simulink model "BALL_BALACING"  (R2021a)
settings: Solver=FixedStepAuto  StartTime=0.0  StopTime=10.0  RelTol=1e-3  EnableMultiTasking=on
libraries: arduinosensorlib x1, arduinolib x1
settings Model: SILPILModeSetting=veronly  ExtModeTrigDuration=2  Creator=Waseem Sajjad  LastModifiedBy=Waseem Sajjad
settings OptimizationCC: EnhancedBackFolding=on  PassReuseOutputArgsAs=Individual arguments  ZeroExternalMemoryAtStartup=off  ZeroInternalMemoryAtStartup=off  MaxStackSize=64  OptimizeBlockOrder=speed  DifferentSizesBufferReuse=on  OptimizationCustomize=off  EfficientTunableParamExpr=on
settings DebuggingCC: ParameterTunabilityLossMsg=error
settings HardwareCC: ProdBitPerInt=16  ProdBitPerPointer=16  ProdBitPerSizeT=16  ProdBitPerPtrDiffT=16  ProdLargestAtomicFloat=None  ProdWordSize=8  ProdHWDeviceType=Atmel->AVR
settings SFSimCC: MATLABDynamicMemAlloc=off
settings RTWCC: SystemTargetFile=ert.tlc  HardwareBoard=Arduino Mega 2560  TemplateMakefile=ert_default_tmf  Toolchain=Arduino AVR  BuildConfiguration=Faster Runs
settings CodeAppCC: ForceParamTrailComments=on  IgnoreCustomStorageClasses=off  OperatorAnnotations=on  SimulinkDataObjDesc=on  SFDataObjDesc=on  InsertBlockDesc=on
settings ERTTargetCC: SupportContinuousTime=on  SupportVariableSizeSignals=on  ExtModeStaticAllocSize=2048

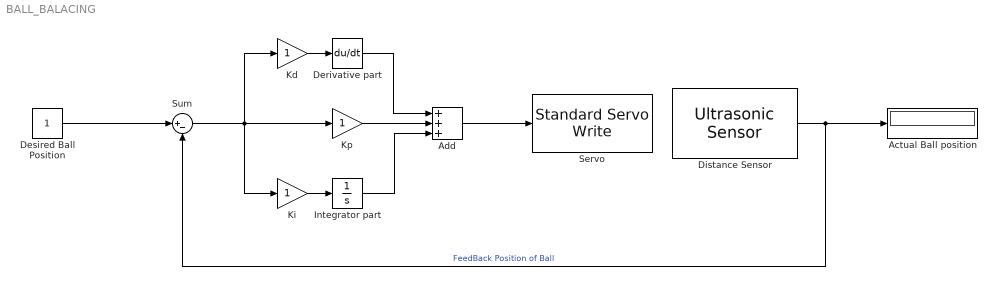
== system BALL_BALACING ==
  Actual Ball position : Display
  Add : Sum  Inputs=+++
  Derivative part : Derivative
  Desired Ball Position : Constant
  Distance Sensor : arduinosensorlib/Ultrasonic Sensor  NumSignalPins=1  TrigPin=4  EchoPin=5  SignalPin=3  SampleTime_=0.1  blockPlatform=ARDUINO
      settings: SourceProductBaseCode=ARDUINO
  Integrator part : Integrator
  Kd : Gain
  Ki : Gain
  Kp : Gain
  Servo : arduinolib/Standard Servo Write  pinNumber=9  ServoIndex=0  blockPlatform=ARDUINO
  Sum : Sum  Inputs=|+-
  wires:
  Kd/1 -> Derivative part/1
  Sum/1 -> Ki/1, Kd/1, Kp/1
  Kp/1 -> Add/2
  Derivative part/1 -> Add/1
  Integrator part/1 -> Add/3
  Add/1 -> Servo/1
  Distance Sensor/1 -> Sum/2, Actual Ball position/1  "FeedBack Position of Ball"
  Desired Ball Position/1 -> Sum/1
  Ki/1 -> Integrator part/1
